simulink model "ExponentialHorn_frequencyResponse"  (Simulink 7.8)
settings: Solver=FixedStepDiscrete  StartTime=0.0  StopTime=1.0  FixedStep=1.0  RelTol=1e-3
undefined symbols (not defined in the file): a_matrix, curvedDuct, d_matrix
settings Model: Creator=emmert  LastModifiedBy=smith

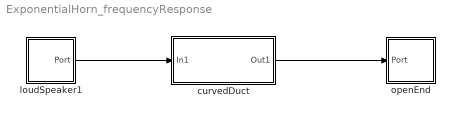
== system ExponentialHorn_frequencyResponse ==
  curvedDuct : Subsystem  mask{surface_poly=exp(2.*x), d_Auto=on, d_polyin='1', l=1, n=25, aj=7.3891}
      mask prompts: surface_poly "Area function A(x) (m²)"; d_Auto "Diameter Automatic"; d_polyin "Diameter function D(x) (m)"; l "Length (m)"; n "Number of "discretization" elements"; aj "Area out (m^2)"
      mask init:
      | switch d_Auto
      |        case 1
      |            d_poly='-1';
      |        case 0 
      |            d_poly=d_polyin;   
      |    end
      |     
      |    tk=0;
      |    
      |   
      |    for kk = -0.5:1:n+1      
      |        tk=tk+1;
      |        xx=kk*l/n ;
      |        x=max(xx,0) ;
      |        x=min(x,l) ; 
      |        Di = double(eval(d_poly)); 
      |        switch d_Auto
      |            case 0
      |             if Di<0
      |                errordlg('diameter must be bigger than or equal to zero','invalid diameter');
      |             end
      |        end
      | 
      |        ai = double(eval(surface_poly));
      |        if ai<=0
      |            errordlg('areas must be positive','invalid areas');
      |        end
      |        d_matrix(tk,1)=Di;
      |        a_matrix(tk,1)=ai;
      |    end
      | 
      |    x = l;
      |    aj = double(eval(surface_poly));
      mask CallbackString:
      | maskStr = get_param(gcb,'MaskValues');
      | x = eval(maskStr{4});
      | a = eval(maskStr{1});
      | maskStr{6} = num2str(a);
      | set_param(gcb,'MaskValues',maskStr);|maskStr = get_param(gcb,'MaskValues');
      | 
      | % check if The checkbox is selected or not.
      | 
      | if strcmp(maskStr{2},'on')
      | 
      |     MaskVisibi=get_param(gcb,'MaskVisibilities');
      |     MaskVisibi{3}='off';
      |     set_param(gcb,'MaskVisibilities',MaskVisibi)
      | else
      |     MaskVisibi=get_param(gcb,'MaskVisibilities');
      |     MaskVisibi{3}='on';
      |     set_param(gcb,'MaskVisibilities',MaskVisibi)
      | end||maskStr = get_param(gcb,'MaskValues');
      | x = eval(maskStr{4});
      | a = eval(maskStr{1});
      | maskStr{6} = num2str(a);
      | set_param(gcb,'MaskValues',maskStr);||
      mask Display:
      | patch([0  .2 .3 .7 .8 1  1  .8 .7 .3 .2  0],...
      |       [.2 .1 .1 .3 .3 .2 .8 .7 .7 .9 .9 .8],[.7 1 1])
      | plot([0 .2 .3 .7 .8 1],[.2 .1 .1 .3 .3 .2])
      | plot([0 .2 .3 .7 .8 1],[.8 .9 .9 .7 .7 .8])
      | text(.4,.5,'A(x)','HorizontalAlignment','center')
      | plot([1 1 0 0 1],[1 0 0 1 1])
  loudSpeaker1 : Subsystem  mask{loc=Upstream, Amp=1, c=100, Mach=0, rho=1, D=sqrt(1/pi), element=loudSpeaker, a=1}
      mask prompts: loc "Location"; Amp "Forcing Amplitude [m/s]"; c "Speed of sound (m/s)"; Mach "Mach number (dimensionless)"; rho "Density (Kg/m³)"; D "Diameter (m)"; a "Area"
      mask init:
      | if Mach<0
      |    errordlg('Mach Number must be bigger than or equal to zero','invalid Mach Number');
      | end
      | 
      | 
      | if c<=0
      |     errordlg('speed of sound must be positive','invalid speed of sound');
      | end
      | 
      | 
      | if D<=0
      |      errordlg('diameter must be positive','invalid diameter');
      | 
      | end
      | 
      | 
      | if rho<=0
      |      errordlg('density must be positive','invalid density');
      | end
      | 
      | % Set identifier
      | set_param(gcb,'element',char('loudSpeaker'));
      | 
      | switchBCUpDownStream(gcb,loc);
      settings: AttributesFormatString=%<Amp> m/s
      mask StyleString: popup(Downstream|Upstream),edit,edit,edit,edit,edit,edit,edit
      mask Display:
      | plot([.2 .2 .4 .4 .2],[.6 .4 .4 .6 .6])
      | plot([.7 .7 .4 .4 .7],[.9 .1 .3 .7 .9])
  openEnd : Subsystem  mask{loc=Downstream, c=100, Mach=0, rho=1.2, D=1, element=openEnd}
      mask prompts: loc "Location"; c "Speed of sound (m/s)"; Mach "Mach number (dimensionless)"; rho "Density (Kg/m³)"; D "Diameter (m)"
      mask init:
      | if Mach<0
      |    errordlg('Mach Number must be bigger than or equal to zero','invalid Mach Number');
      | end
      | 
      | 
      | if c<=0
      |     errordlg('speed of sound must be positive','invalid speed of sound');
      | end
      | 
      | 
      | if D<=0
      |      errordlg('diameter must be positive','invalid diameter');
      | 
      | end
      | 
      | 
      | if rho<=0
      |      errordlg('density must be positive','invalid density');
      | end
      | 
      | % Set identifier
      | set_param(gcb,'element',char('openEnd'));
      | 
      | switchBCUpDownStream(gcb,loc);
      mask StyleString: popup(Downstream|Upstream),edit,edit,edit,edit,edit
      mask Display:
      | %patch([.2  1  1 .2],[.2 .2 .8 .8],[.7 1 1])
      | %patch([.2 .3 .3 .2],[.2 .2 .8 .8],[.9 1 1])
      | %patch([.3 .4 .4 .3],[.2 .2 .8 .8],[.8 1 1])
      | %plot([.3 1],[.2 .2])
      | %plot([.3 1],[.8 .8])
      | %plot([1 1 0 0 1],[1 0 0 1 1])
      | 
      | %patch([.2 .2 .3 .5 .6 .6 .5 .3],...
      | %      [.45 .65 .75 .75 .65 .45 .35 .35],[1 1 0])
      | color('red')
      | plot([.25 .2  .2  .3  .5  .6  .6],...
      |      [.4  .45 .65 .75 .75 .65 .5])
      | plot([.4 .4],[.85 1.0])
      | plot([-.05 .1],[.55 .55])
      | plot([.7 .85],[.55 .55])
      | plot([.2 .1],[.75 .85])
      | plot([.6 .7],[.75 .85])
      | %patch([.1 .1 .2 .4 .45 .6 .75 .9  .9 1. 1. .9 .2],...
      | %      [.1 .3 .4 .4 .35 .5  .5 .35 .3 .2 .1 .0 .0],[.7 1 1])
      | color('blue')
      | plot([ .45 .6 .75 .9  .9 1. 1. .9 .2 .1 .1 .2 .4 .6 .7],...
      |      [ .35 .5  .5 .35 .3 .2 .1 .0 .0 .1 .3 .4 .4 .2 .2])
  wires:
  loudSpeaker1/1(Port) -> curvedDuct/1(In1)
  curvedDuct/1(Out1) -> openEnd/1(Port)

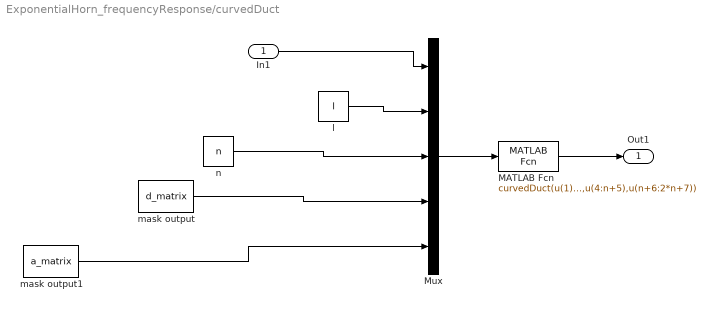
== system ExponentialHorn_frequencyResponse/curvedDuct ==
  In1 : Inport
  MATLAB Fcn : MATLABFcn  MATLABFcn=curvedDuct(u(1),u(2),u(3),u(4:n+5),u(n+6:2*n+7))  OutputDimensions=1
  Mux : Mux  Inputs=5
  l : Constant  Value=l
  mask output : Constant  Value=d_matrix
  mask output1 : Constant  Value=a_matrix
  n : Constant  Value=n
  Out1 : Outport
  wires:
  In1/1 -> Mux/1
  Mux/1 -> MATLAB Fcn/1
  MATLAB Fcn/1 -> Out1/1
  l/1 -> Mux/2
  n/1 -> Mux/3
  mask output/1 -> Mux/4
  mask output1/1 -> Mux/5

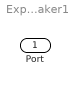
== system ExponentialHorn_frequencyResponse/loudSpeaker1 ==
  Port : Outport

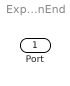
== system ExponentialHorn_frequencyResponse/openEnd ==
  Port : Inport
